simulink model "HVDC_VSC_1CPUcore_dcpl"  (Simulink 8.4)
settings: Solver=ode3  SolverMode=SingleTasking  StartTime=0.0  StopTime=70.0  FixedStep=Ts_Power  RelTol=1e-3  AbsTol=1e-2
PreLoadFcn:
  | Ts_Power=50e-6; Ts_Control=1*Ts_Power; init_cosim_IA; startup_transients_hvdc_vsc;
PostLoadFcn:
  | Ts_Power=50e-6; Ts_Control=1*Ts_Power; init_cosim_IA; startup_transients_hvdc_vsc;
InitFcn:
  | Ts_Power=50e-6; Ts_Control=1*Ts_Power; init_cosim_IA; startup_transients_hvdc_vsc;
values from neighbouring files (symbols this model uses):
  dPref1_2 = 0.125    [startup_transients_hvdc_vsc.m]
  dPref1_2_rlimit = 0.6    [startup_transients_hvdc_vsc.m]
  t_deblock_Pref1 = 0.5    [startup_transients_hvdc_vsc.m]
  t_deblock_Udref2 = 0.3    [startup_transients_hvdc_vsc.m]
  t_dPref1_2 = 25.0    (= 25)    [startup_transients_hvdc_vsc.m]
  t_SwitchITMIdc = 0.2    [startup_transients_hvdc_vsc.m]
  t_SwitchITMVdc = 0.1    [startup_transients_hvdc_vsc.m]
undefined symbols (not defined in the file or in its folder): CLARK, D1, Delta, gcbh, h, intfDelay, level, lib_mesures, magnitude, ResistanceM, rte_drive_private_lib, rte_tsb3level_hiz_rect_cb, sps_rtmsupport, Ts_intf, TSB3_hiZR
libraries: powerlib x183, spsVIMeasurementModel x102, powerlib_extras x71, powerlib_meascontrol x50, rteventslib x26, op_dpl_lib x20, rtlab x12, sps_avr x6, artemis x1
(part 1 of 13)
Description:
  | The 'Model  initialization function' defined in the
  | 
  | Model Properties automatically sets the sample time
  | 
  | Ts to 50e-6 s
settings Model: ARTEMISmethode_block_infos=$$__separator__$$HVDC_VSC_1CPUcore_dcpl/ARTEMIS Guide$$__separator__$$  Creator=Gilbert Sybille, IREQ  LastModifiedBy=marij  CovSFcnEnable=on  ExtModeTrigMode=oneshot  ExtModeArmWhenConnect=off  ExtModeAutoUpdateStatusClock=off  BufferReuse=off
settings DataIOCC: LimitDataPoints=off  SaveFormat=StructureWithTime  SaveOutput=off  DSMLogging=off  SaveTime=off  SignalLoggingName=sigsOut
settings OptimizationCC: BlockReduction=off  BooleanDataType=off  OptimizeBlockIOStorage=off  BufferReuse=off  GlobalBufferReuse=off  ExpressionFolding=off  LocalBlockOutputs=off  InitFltsAndDblsToZero=on
settings DebuggingCC: SaveWithParameterizedLinksMsg=none  CheckExecutionContextPreStartOutputMsg=on  CheckExecutionContextRuntimeOutputMsg=on  SignalResolutionControl=TryResolveAllWithWarning  SolverPrmCheckMsg=none  MultiTaskDSMMsg=warning  MultiTaskCondExecSysMsg=none  FcnCallInpInsideContextMsg=EnableAllAsWarning  UnconnectedInputMsg=none  UnconnectedOutputMsg=none  UnconnectedLineMsg=none  FrameProcessingCompatibilityMsg=error
settings HardwareCC: TargetHWDeviceType=32-bit Generic  ProdEqTarget=off
settings GRTTargetCC: TargetFcnLib=ansi_tfl_tmw.mat

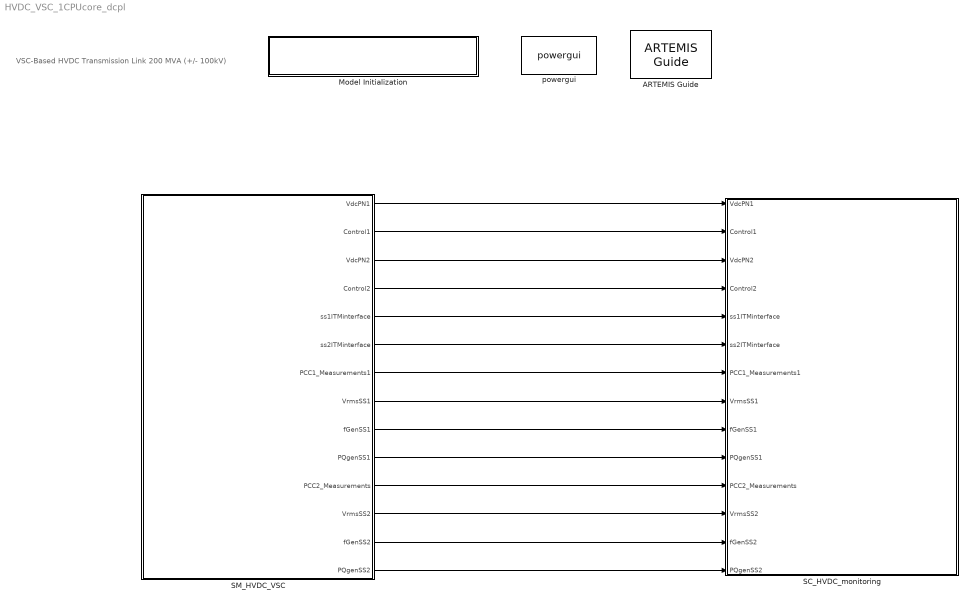
== system HVDC_VSC_1CPUcore_dcpl ==
  note: VSC-Based HVDC Transmission Link
      | 200 MVA  (+/- 100kV)
  ARTEMIS Guide : artemis/ARTEMIS/ARTEMIS Guide  Tag=FTSSmethode_opal_4hx0r99  Description=5.0_z1  lock=on  Ts=Ts_Power  opt=art5  dyna=off  nb_perm=4  RT_fullcomp=off  ssn=off  ssn_itvc=off  ssn_ivic=off  ssn_ext=off  ssn_solver=Trapezoidal  ssn_impulse=off  ssn_quasimpulse=off  ssn_impulse_loop=5  paraExtinctionThy=off  Thy_Impulse=on  dtc=Off  dtc_opt=normal  ao=on  simtype=off  ct_mac=off  lin_mov=off  lsp=[0.001 2]  spike_skip=Disabled  dtc_extra=1  dtc_sws=normal  dtc_pied=0.5  SPSRulesBlock=SPSRules  tre=on  ctmm=off  LF=off  dpl_type=ARTEMiS DPL  rlc_type=off  custom_type=off  para=on  ssn_ImpulseLoopBlockedStateUpdate=5  ssn_mov_iter_number=5  ssn_switch_iter_number=5
  Model Initialization : Subsystem  mask(Model Functions){InitFcnX=Ts_Power=50e-6; Ts_Control=1*Ts_Power; init_cosim_IA; startup_transients_hvdc_vsc;, prel=on, posl=on, inif=on, strf=off}
      mask prompts: InitFcnX "Initialisation"; prel "Preload Function"; posl "PostLoad Function"; inif "InitFcn"; strf "StartFcn"
      mask init:
      | currentBlock = gcb;
      | root = bdroot(currentBlock);
      | 
      | if ~strcmp(get_param(root,'BlockDiagramType'),'library')
      |     if prel==1
      |         set_param(root, 'PreLoadFcn', InitFcnX);
      |     else
      |         set_param(root, 'PreLoadFcn', '');
      |     end
      |     if inif==1
      |         set_param(root, 'InitFcn', InitFcnX);
      |     else
      |         set_param(root, 'InitFcn', '');
      |     end
      |     if strf==1
      |         set_param(root, 'StartFcn', InitFcnX);
      |     else
      |         set_param(root, 'StartFcn', '');
      |     end
      |     if posl==1
      |         set_param(root, 'PostLoadFcn', InitFcnX);
      |     else
      |         set_param(root, 'PostLoadFcn', '');
      |     end
      | end
      | 
      | pos = get_param(currentBlock, 'Position');
      | width = pos(3) - pos(1); height = pos(4) - pos(2);
      | txt = [ upper(root) '\n' '- InitFcn. . . . . '  get_param(root, 'InitFcn') ];
      settings: CopyFcn=set_param(gcb,'LinkStatus','none')
      mask Display: text(5, height*0.5, txt, 'horizontalAlignment', 'left', 'verticalAlignment', 'middle') ;
  SC_HVDC_monitoring : Subsystem
  SM_HVDC_VSC : Subsystem
  powergui : powerlib/powergui  Priority=2  SimulationMode=Discrete  SolverType=Tustin  SampleTime=Ts_Power  frequency=60  SPID=off  DisableSnubberDevices=off  DisableRonSwitches=off  DisableVfSwitches=off  SwTol=0  DisplayEquations=off  Interpol=off  methode=off  Ts=0  frequencyindice=0  Pbase=100e6  ErrMax=1e-4  Iterations=50  UnitsV=kV  UnitsW=MW  FunctionMessages=off  echomessages=on  HookPort=off  EnableUseOfTLC=off  x0status=zero  RestoreLinks=warning  ResistiveCurrentMeasurement=off  Frange=[0:2:500]  Ylog=off  Xlog=on  ShowGrid=off  save=off  variable=ZData  structure=res_fft  ZoomFFT=on  StartTime=1.5  cycles=2  DisplayStyle=1  fundamental=50  FreqAxis=off  MaxFrequency=3000  frequencyindicesteady=1  RmsSteady=1  display=off
  wires:
  SM_HVDC_VSC/1(VdcPN1) -> SC_HVDC_monitoring/1(VdcPN1)
  SM_HVDC_VSC/2(Control1) -> SC_HVDC_monitoring/2(Control1)
  SM_HVDC_VSC/3(VdcPN2) -> SC_HVDC_monitoring/3(VdcPN2)
  SM_HVDC_VSC/4(Control2) -> SC_HVDC_monitoring/4(Control2)
  SM_HVDC_VSC/5(ss1ITMinterface) -> SC_HVDC_monitoring/5(ss1ITMinterface)
  SM_HVDC_VSC/6(ss2ITMinterface) -> SC_HVDC_monitoring/6(ss2ITMinterface)
  SM_HVDC_VSC/11(PCC2_Measurements) -> SC_HVDC_monitoring/11(PCC2_Measurements)
  SM_HVDC_VSC/13(fGenSS2) -> SC_HVDC_monitoring/13(fGenSS2)
  SM_HVDC_VSC/7(PCC1_Measurements1) -> SC_HVDC_monitoring/7(PCC1_Measurements1)
  SM_HVDC_VSC/8(VrmsSS1) -> SC_HVDC_monitoring/8(VrmsSS1)
  SM_HVDC_VSC/14(PQgenSS2) -> SC_HVDC_monitoring/14(PQgenSS2)
  SM_HVDC_VSC/10(PQgenSS1) -> SC_HVDC_monitoring/10(PQgenSS1)
  SM_HVDC_VSC/9(fGenSS1) -> SC_HVDC_monitoring/9(fGenSS1)
  SM_HVDC_VSC/12(VrmsSS2) -> SC_HVDC_monitoring/12(VrmsSS2)

== system HVDC_VSC_1CPUcore_dcpl/Model Initialization ==

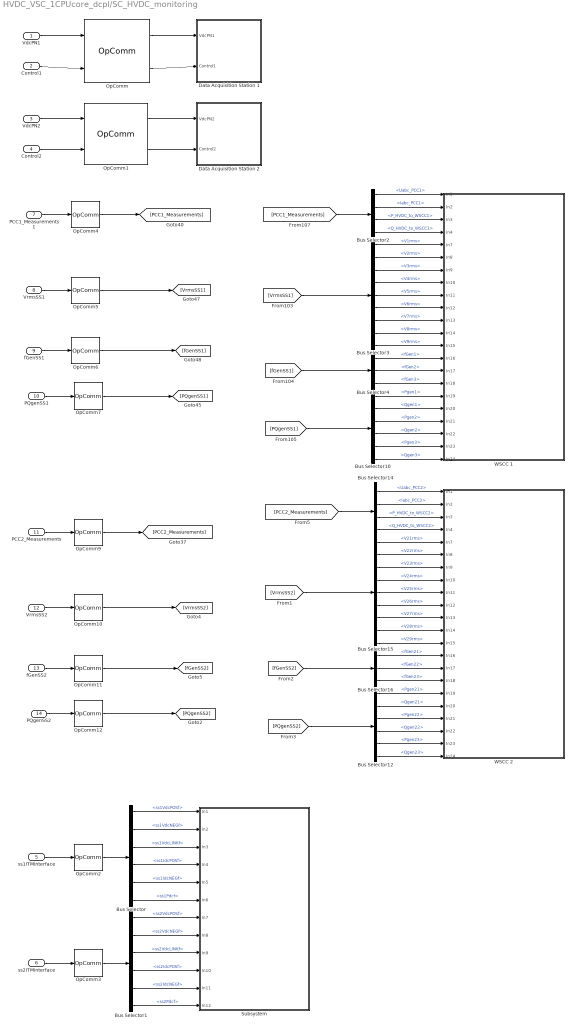
== system HVDC_VSC_1CPUcore_dcpl/SC_HVDC_monitoring ==
  VdcPN1 : Inport
  Control1 : Inport  Port=2
  VdcPN2 : Inport  Port=3
  Control2 : Inport  Port=4
  ss1ITMinterface : Inport  Port=5
  ss2ITMinterface : Inport  Port=6
  PCC1_Measurements1 : Inport  Port=7
  VrmsSS1 : Inport  Port=8
  fGenSS1 : Inport  Port=9
  PQgenSS1 : Inport  Port=10
  PCC2_Measurements : Inport  Port=11
  VrmsSS2 : Inport  Port=12
  fGenSS2 : Inport  Port=13
  PQgenSS2 : Inport  Port=14
  Bus Selector : BusSelector  OutputSignals=ss1VdcPOSf,ss1VdcNEGf,ss1VdcLINKf,ss1IdcPOSf,ss1IdcNEGf,ss1Pdcf
  Bus Selector1 : BusSelector  OutputSignals=ss2VdcPOSf,ss2VdcNEGf,ss2VdcLINKf,ss2IdcPOSf,ss2IdcNEGf,ss2Pdcf
  Bus Selector10 : BusSelector  OutputSignals=Pgen1,Qgen1,Pgen2,Qgen2,Pgen3,Qgen3
  Bus Selector12 : BusSelector  OutputSignals=Pgen21,Qgen21,Pgen22,Qgen22,Pgen23,Qgen23
  Bus Selector14 : BusSelector  OutputSignals=Uabc_PCC2,Iabc_PCC2,P_HVDC_to_WSCC2,Q_HVDC_to_WSCC2
  Bus Selector15 : BusSelector  OutputSignals=V21rms,V22rms,V23rms,V24rms,V25rms,V26rms,V27rms,V28rms,V29rms
  Bus Selector16 : BusSelector  OutputSignals=fGen21,fGen22,fGen23
  Bus Selector2 : BusSelector  OutputSignals=Uabc_PCC1,Iabc_PCC1,P_HVDC_to_WSCC1,Q_HVDC_to_WSCC1
  Bus Selector3 : BusSelector  OutputSignals=V1rms,V2rms,V3rms,V4rms,V5rms,V6rms,V7rms,V8rms,V9rms
  Bus Selector4 : BusSelector  OutputSignals=fGen1,fGen2,fGen3
  Data Acquisition Station 1 : Subsystem
      mask Display: disp('Open this block\nto visualize\nrecorded signals')
  Data Acquisition Station 2 : Subsystem
      mask Display: disp('Open this block\nto visualize\nrecorded signals')
  OpComm : rtlab/OpComm  nbport=2  groupe_acq=1  subsys_rate=Ts_Power  st=0  Synchronization=on  Interpolation=on  Threshold=1.0  Missed_Data=off  Sim_Time=off  Samples=off  dynSigOut=off  from_console=0  warning_done=off  writeOpCommFile=off  Offset=off
  OpComm1 : rtlab/OpComm  nbport=2  groupe_acq=2  subsys_rate=Ts_Power  st=0  Synchronization=on  Interpolation=on  Threshold=1.0  Missed_Data=off  Sim_Time=off  Samples=off  dynSigOut=off  from_console=0  warning_done=off  writeOpCommFile=off  Offset=off
  OpComm10 : rtlab/OpComm  nbport=1  groupe_acq=10  subsys_rate=Ts_Power  st=0  Synchronization=on  Interpolation=on  Threshold=1.0  Missed_Data=off  Sim_Time=off  Samples=off  dynSigOut=off  from_console=0  warning_done=off  writeOpCommFile=off  Offset=off
  OpComm11 : rtlab/OpComm  nbport=1  groupe_acq=11  subsys_rate=Ts_Power  st=0  Synchronization=on  Interpolation=on  Threshold=1.0  Missed_Data=off  Sim_Time=off  Samples=off  dynSigOut=off  from_console=0  warning_done=off  writeOpCommFile=off  Offset=off
  OpComm12 : rtlab/OpComm  nbport=1  groupe_acq=12  subsys_rate=Ts_Power  st=0  Synchronization=on  Interpolation=on  Threshold=1.0  Missed_Data=off  Sim_Time=off  Samples=off  dynSigOut=off  from_console=0  warning_done=off  writeOpCommFile=off  Offset=off
  OpComm2 : rtlab/OpComm  nbport=1  groupe_acq=3  subsys_rate=Ts_Power  st=0  Synchronization=on  Interpolation=on  Threshold=1.0  Missed_Data=off  Sim_Time=off  Samples=off  dynSigOut=off  from_console=0  warning_done=off  writeOpCommFile=off  Offset=off
  OpComm3 : rtlab/OpComm  nbport=1  groupe_acq=4  subsys_rate=Ts_Power  st=0  Synchronization=on  Interpolation=on  Threshold=1.0  Missed_Data=off  Sim_Time=off  Samples=off  dynSigOut=off  from_console=0  warning_done=off  writeOpCommFile=off  Offset=off
  OpComm4 : rtlab/OpComm  nbport=1  groupe_acq=5  subsys_rate=Ts_Power  st=0  Synchronization=on  Interpolation=on  Threshold=1.0  Missed_Data=off  Sim_Time=off  Samples=off  dynSigOut=off  from_console=0  warning_done=off  writeOpCommFile=off  Offset=off
  OpComm5 : rtlab/OpComm  nbport=1  groupe_acq=6  subsys_rate=Ts_Power  st=0  Synchronization=on  Interpolation=on  Threshold=1.0  Missed_Data=off  Sim_Time=off  Samples=off  dynSigOut=off  from_console=0  warning_done=off  writeOpCommFile=off  Offset=off
  OpComm6 : rtlab/OpComm  nbport=1  groupe_acq=7  subsys_rate=Ts_Power  st=0  Synchronization=on  Interpolation=on  Threshold=1.0  Missed_Data=off  Sim_Time=off  Samples=off  dynSigOut=off  from_console=0  warning_done=off  writeOpCommFile=off  Offset=off
  OpComm7 : rtlab/OpComm  nbport=1  groupe_acq=8  subsys_rate=Ts_Power  st=0  Synchronization=on  Interpolation=on  Threshold=1.0  Missed_Data=off  Sim_Time=off  Samples=off  dynSigOut=off  from_console=0  warning_done=off  writeOpCommFile=off  Offset=off
  OpComm9 : rtlab/OpComm  nbport=1  groupe_acq=9  subsys_rate=Ts_Power  st=0  Synchronization=on  Interpolation=on  Threshold=1.0  Missed_Data=off  Sim_Time=off  Samples=off  dynSigOut=off  from_console=0  warning_done=off  writeOpCommFile=off  Offset=off
  Subsystem : Subsystem
  WSCC 1 : Subsystem
  WSCC 2 : Subsystem
  wires:
  VdcPN1/1 -> OpComm/1
  Control1/1 -> OpComm/2
  OpComm/1 -> Data Acquisition Station 1/1(VdcPN1)
  OpComm/2 -> Data Acquisition Station 1/2(Control1)
  VdcPN2/1 -> OpComm1/1
  Control2/1 -> OpComm1/2
  OpComm1/1 -> Data Acquisition Station 2/1(VdcPN2)
  OpComm1/2 -> Data Acquisition Station 2/2(Control2)
  ss1ITMinterface/1 -> OpComm2/1
  OpComm2/1 -> Bus Selector/1
  ss2ITMinterface/1 -> OpComm3/1
  OpComm3/1 -> Bus Selector1/1
  Bus Selector/1 -> Subsystem/1(In1)  "<ss1VdcPOSf>"
  Bus Selector/2 -> Subsystem/2(In2)  "<ss1VdcNEGf>"
  Bus Selector/3 -> Subsystem/3(In3)  "<ss1VdcLINKf>"
  Bus Selector/4 -> Subsystem/4(In4)  "<ss1IdcPOSf>"
  Bus Selector/5 -> Subsystem/5(In5)  "<ss1IdcNEGf>"
  Bus Selector/6 -> Subsystem/6(In6)  "<ss1Pdcf>"
  Bus Selector1/1 -> Subsystem/7(In7)  "<ss2VdcPOSf>"
  Bus Selector1/2 -> Subsystem/8(In8)  "<ss2VdcNEGf>"
  Bus Selector1/3 -> Subsystem/9(In9)  "<ss2VdcLINKf>"
  Bus Selector1/4 -> Subsystem/10(In10)  "<ss2IdcPOSf>"
  Bus Selector1/5 -> Subsystem/11(In11)  "<ss2IdcNEGf>"
  Bus Selector1/6 -> Subsystem/12(In12)  "<ss2Pdcf>"
  [PCC1_Measurements] -> Bus Selector2/1
  [VrmsSS1] -> Bus Selector3/1
  [fGenSS1] -> Bus Selector4/1
  [PQgenSS1] -> Bus Selector10/1
  PCC1_Measurements1/1 -> OpComm4/1
  VrmsSS1/1 -> OpComm5/1
  fGenSS1/1 -> OpComm6/1
  PQgenSS1/1 -> OpComm7/1
  OpComm4/1 -> [PCC1_Measurements]
  OpComm5/1 -> [VrmsSS1]
  OpComm6/1 -> [fGenSS1]
  OpComm7/1 -> [PQgenSS1]
  Bus Selector2/1 -> WSCC 1/1(In1)  "<Uabc_PCC1>"
  Bus Selector2/2 -> WSCC 1/2(In2)  "<Iabc_PCC1>"
  Bus Selector2/3 -> WSCC 1/3(In3)  "<P_HVDC_to_WSCC1>"
  Bus Selector2/4 -> WSCC 1/4(In4)  "<Q_HVDC_to_WSCC1>"
  Bus Selector3/1 -> WSCC 1/5(In7)  "<V1rms>"
  Bus Selector3/2 -> WSCC 1/6(In8)  "<V2rms>"
  Bus Selector3/3 -> WSCC 1/7(In9)  "<V3rms>"
  Bus Selector3/4 -> WSCC 1/8(In10)  "<V4rms>"
  Bus Selector3/5 -> WSCC 1/9(In11)  "<V5rms>"
  Bus Selector3/6 -> WSCC 1/10(In12)  "<V6rms>"
  Bus Selector3/7 -> WSCC 1/11(In13)  "<V7rms>"
  Bus Selector3/8 -> WSCC 1/12(In14)  "<V8rms>"
  Bus Selector3/9 -> WSCC 1/13(In15)  "<V9rms>"
  Bus Selector4/1 -> WSCC 1/14(In16)  "<fGen1>"
  Bus Selector4/2 -> WSCC 1/15(In17)  "<fGen2>"
  Bus Selector4/3 -> WSCC 1/16(In18)  "<fGen3>"
  Bus Selector10/1 -> WSCC 1/17(In19)  "<Pgen1>"
  Bus Selector10/2 -> WSCC 1/18(In20)  "<Qgen1>"
  Bus Selector10/3 -> WSCC 1/19(In21)  "<Pgen2>"
  Bus Selector10/4 -> WSCC 1/20(In22)  "<Qgen2>"
  Bus Selector10/5 -> WSCC 1/21(In23)  "<Pgen3>"
  Bus Selector10/6 -> WSCC 1/22(In24)  "<Qgen3>"
  [PCC2_Measurements] -> Bus Selector14/1
  [VrmsSS2] -> Bus Selector15/1
  [fGenSS2] -> Bus Selector16/1
  [PQgenSS2] -> Bus Selector12/1
  PCC2_Measurements/1 -> OpComm9/1
  VrmsSS2/1 -> OpComm10/1
  fGenSS2/1 -> OpComm11/1
  PQgenSS2/1 -> OpComm12/1
  OpComm9/1 -> [PCC2_Measurements]
  OpComm10/1 -> [VrmsSS2]
  OpComm11/1 -> [fGenSS2]
  OpComm12/1 -> [PQgenSS2]
  Bus Selector14/1 -> WSCC 2/1(In1)  "<Uabc_PCC2>"
  Bus Selector14/2 -> WSCC 2/2(In2)  "<Iabc_PCC2>"
  Bus Selector14/3 -> WSCC 2/3(In3)  "<P_HVDC_to_WSCC2>"
  Bus Selector15/2 -> WSCC 2/6(In8)  "<V22rms>"
  Bus Selector15/3 -> WSCC 2/7(In9)  "<V23rms>"
  Bus Selector15/5 -> WSCC 2/9(In11)  "<V25rms>"
  Bus Selector15/7 -> WSCC 2/11(In13)  "<V27rms>"
  Bus Selector15/8 -> WSCC 2/12(In14)  "<V28rms>"
  Bus Selector15/9 -> WSCC 2/13(In15)  "<V29rms>"
  Bus Selector16/1 -> WSCC 2/14(In16)  "<fGen21>"
  Bus Selector16/2 -> WSCC 2/15(In17)  "<fGen22>"
  Bus Selector16/3 -> WSCC 2/16(In18)  "<fGen23>"
  Bus Selector12/1 -> WSCC 2/17(In19)  "<Pgen21>"
  Bus Selector12/2 -> WSCC 2/18(In20)  "<Qgen21>"
  Bus Selector12/3 -> WSCC 2/19(In21)  "<Pgen22>"
  Bus Selector12/4 -> WSCC 2/20(In22)  "<Qgen22>"
  Bus Selector12/5 -> WSCC 2/21(In23)  "<Pgen23>"
  Bus Selector12/6 -> WSCC 2/22(In24)  "<Qgen23>"
  Bus Selector15/4 -> WSCC 2/8(In10)  "<V24rms>"
  Bus Selector15/6 -> WSCC 2/10(In12)  "<V26rms>"
  Bus Selector14/4 -> WSCC 2/4(In4)  "<Q_HVDC_to_WSCC2>"
  Bus Selector15/1 -> WSCC 2/5(In7)  "<V21rms>"

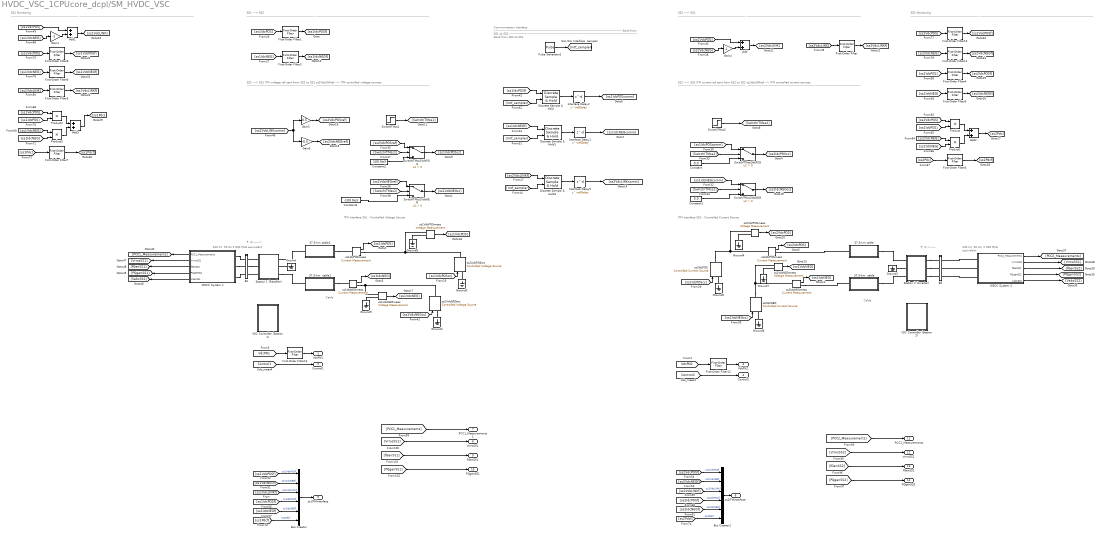
== system HVDC_VSC_1CPUcore_dcpl/SM_HVDC_VSC ==
  note: 230 kV, 50 Hz
      |  2 000 MVA equivalent
  note: P, Q
      | <------
  note: P, Q
      | ------>
  note: Cable
  note: 230 kV, 50 Hz,
      | 2 000 MVA equivalent
  note: Cable
  note: SS2 ---> SS1
      | ITM voltage ref sent from SS2 to SS1
      | ss2VdcLINKref
      | --> ITM controlled voltage sources
      | ------------------------------------------------------------------------------------------------------------------------------------------------------------------------------------
  note: Communication Interface
      |
      | --------------------------------------------------------------------------------------------------------------------------------
      | Send from SS1 to SS2
      |
      | --------------------------------------------------------------------------------------------------------------------------------
      | Send from SS2 to SS1
  note: SS1 ---> SS2
      | ------------------------------------------------------------------------------------------------------------------------------------------------------------------------------------
  note: SS2 ---> SS1
      | ------------------------------------------------------------------------------------------------------------------------------------------------------------------------------------
  note: SS1 ---> SS2
      | ITM current ref sent from SS1 to SS2
      | ss1IdcLINKref
      | --> ITM controlled current sources
      | ------------------------------------------------------------------------------------------------------------------------------------------------------------------------------------
  note: ITM Interface SS1 - Controlled Voltage Source
  note: ITM Interface SS2 - Controlled Current Source
  note: SS1 Monitoring
      | ------------------------------------------------------------------------------------------------------------------------------------------------------------------------------------
  note: SS2 Monitoring
      | ------------------------------------------------------------------------------------------------------------------------------------------------------------------------------------
  37.5-km  cable : Subsystem  mask(Artemis Distributed Parameters Line){SimulationMode=ARTEMIS model, Phases=1, Frequency=60, Resistance=1.3900e-002, Inductance=1.5900e-004, Capacitance=2.3100e-007, Length=37.5, Measurements=None}
      mask prompts: SimulationMode "Simulation Mode"; Phases "Number of phases N"; Frequency "Frequency used for R L C specification (Hz)"; Resistance "Resistance per unit length (Ohms/km)   [N*N matrix] or [R1 R0 R0m]"; Inductance "Inductance per unit length (H/km) [N*N matrix ] or [L1 L0 L0m]"; Capacitance "Capacitance per unit length (F/km) [N*N matrix] or [C1 C0 C0m]"; Length "Line length (km)"
      mask help:
      | Implements a N-phases distributed parameter line model. The R,L, and C line parameters are specified by [NxN] matrices.
      |
      | To model a two-, three-, or a six-phase symetrical line you can either specify complete [NxN] matrices or simply enter sequence parameters vectors: the  positive and zero sequence parameters for a two-phase or  three-phase transposed  line, plus the mutual zero-sequence for a  six-phase transposed  line  (2 coupled 3-phase lines).
      mask init:
      | % Get current block
      | currentBlock = gcb;
      | 
      | % Get electric variables
      | [Zm,R,v,Ti,to,Rt4,h,Zimp,Zmat,Yphase,ResistanceM] = op_distributedparametersline_cb(gcb,'variable_mask_maskinitialization', Phases, Frequency, Resistance, Inductance, Capacitance, Length);
      | 
      | % Set block contents
      | op_distributedparametersline_cb(currentBlock,'maskinitialization');
      mask Help: eval('fts2help(''distributedparametersline'');');
      mask TypeOptions SimulationMode: SimPowerSystems model | ARTEMIS model
      mask TypeOptions Phases: 1 | 2 | 3 | 4 | 5 | 6
      mask TypeOptions Measurements: None
      mask Display:
      | patch([0 0.5 0.7 0],[1 1 0 0],[0.7 0.75 0.9]);
      | patch([1 0.53 0.73 1],[1 1 0 0],[1 0.8 0.7]);
      | plot([0 0 1 1 0],[0 1 1 0 0]);
      | plot([0 0.2 0.2 0.8 0.8 1 0.8 0.8 0.2 0.2 NaN 0 NaN 1],[0.5 0.5 0.625 0.625 0.5 0.5 0.5 0.375 0.375 0.5 NaN 0 NaN 1])
      | disp('DPL')
  37.5-km  cable1 : Subsystem  mask(Artemis Distributed Parameters Line){SimulationMode=ARTEMIS model, Phases=1, Frequency=60, Resistance=1.3900e-002, Inductance=1.5900e-004, Capacitance=2.3100e-007, Length=37.5, Measurements=None}
      mask prompts: SimulationMode "Simulation Mode"; Phases "Number of phases N"; Frequency "Frequency used for R L C specification (Hz)"; Resistance "Resistance per unit length (Ohms/km)   [N*N matrix] or [R1 R0 R0m]"; Inductance "Inductance per unit length (H/km) [N*N matrix ] or [L1 L0 L0m]"; Capacitance "Capacitance per unit length (F/km) [N*N matrix] or [C1 C0 C0m]"; Length "Line length (km)"
      mask help:
      | Implements a N-phases distributed parameter line model. The R,L, and C line parameters are specified by [NxN] matrices.
      |
      | To model a two-, three-, or a six-phase symetrical line you can either specify complete [NxN] matrices or simply enter sequence parameters vectors: the  positive and zero sequence parameters for a two-phase or  three-phase transposed  line, plus the mutual zero-sequence for a  six-phase transposed  line  (2 coupled 3-phase lines).
      mask init: same as HVDC_VSC_1CPUcore_dcpl/SM_HVDC_VSC/37.5-km  cable
      mask Help: eval('fts2help(''distributedparametersline'');');
      mask TypeOptions SimulationMode: SimPowerSystems model | ARTEMIS model
      mask TypeOptions Phases: 1 | 2 | 3 | 4 | 5 | 6
      mask TypeOptions Measurements: None
      mask Display:
      | patch([0 0.5 0.7 0],[1 1 0 0],[0.7 0.75 0.9]);
      | patch([1 0.53 0.73 1],[1 1 0 0],[1 0.8 0.7]);
      | plot([0 0 1 1 0],[0 1 1 0 0]);
      | plot([0 0.2 0.2 0.8 0.8 1 0.8 0.8 0.2 0.2 NaN 0 NaN 1],[0.5 0.5 0.625 0.625 0.5 0.5 0.5 0.375 0.375 0.5 NaN 0 NaN 1])
      | disp('DPL')
  37.5-km cable : Subsystem  mask(Artemis Distributed Parameters Line){SimulationMode=ARTEMIS model, Phases=1, Frequency=60, Resistance=1.3900e-002, Inductance=1.5900e-004, Capacitance=2.3100e-007, Length=37.5, Measurements=None}
      mask prompts: SimulationMode "Simulation Mode"; Phases "Number of phases N"; Frequency "Frequency used for R L C specification (Hz)"; Resistance "Resistance per unit length (Ohms/km)   [N*N matrix] or [R1 R0 R0m]"; Inductance "Inductance per unit length (H/km) [N*N matrix ] or [L1 L0 L0m]"; Capacitance "Capacitance per unit length (F/km) [N*N matrix] or [C1 C0 C0m]"; Length "Line length (km)"
      mask help:
      | Implements a N-phases distributed parameter line model. The R,L, and C line parameters are specified by [NxN] matrices.
      |
      | To model a two-, three-, or a six-phase symetrical line you can either specify complete [NxN] matrices or simply enter sequence parameters vectors: the  positive and zero sequence parameters for a two-phase or  three-phase transposed  line, plus the mutual zero-sequence for a  six-phase transposed  line  (2 coupled 3-phase lines).
      mask init: same as HVDC_VSC_1CPUcore_dcpl/SM_HVDC_VSC/37.5-km  cable
      mask Help: eval('fts2help(''distributedparametersline'');');
      mask TypeOptions SimulationMode: SimPowerSystems model | ARTEMIS model
      mask TypeOptions Phases: 1 | 2 | 3 | 4 | 5 | 6
      mask TypeOptions Measurements: None
      mask Display:
      | patch([0 0.5 0.7 0],[1 1 0 0],[0.7 0.75 0.9]);
      | patch([1 0.53 0.73 1],[1 1 0 0],[1 0.8 0.7]);
      | plot([0 0 1 1 0],[0 1 1 0 0]);
      | plot([0 0.2 0.2 0.8 0.8 1 0.8 0.8 0.2 0.2 NaN 0 NaN 1],[0.5 0.5 0.625 0.625 0.5 0.5 0.5 0.375 0.375 0.5 NaN 0 NaN 1])
      | disp('DPL')
  37.5-km cable1 : Subsystem  mask(Artemis Distributed Parameters Line){SimulationMode=ARTEMIS model, Phases=1, Frequency=60, Resistance=1.3900e-002, Inductance=1.5900e-004, Capacitance=2.3100e-007, Length=37.5, Measurements=None}
      mask prompts: SimulationMode "Simulation Mode"; Phases "Number of phases N"; Frequency "Frequency used for R L C specification (Hz)"; Resistance "Resistance per unit length (Ohms/km)   [N*N matrix] or [R1 R0 R0m]"; Inductance "Inductance per unit length (H/km) [N*N matrix ] or [L1 L0 L0m]"; Capacitance "Capacitance per unit length (F/km) [N*N matrix] or [C1 C0 C0m]"; Length "Line length (km)"
      mask help:
      | Implements a N-phases distributed parameter line model. The R,L, and C line parameters are specified by [NxN] matrices.
      |
      | To model a two-, three-, or a six-phase symetrical line you can either specify complete [NxN] matrices or simply enter sequence parameters vectors: the  positive and zero sequence parameters for a two-phase or  three-phase transposed  line, plus the mutual zero-sequence for a  six-phase transposed  line  (2 coupled 3-phase lines).
      mask init: same as HVDC_VSC_1CPUcore_dcpl/SM_HVDC_VSC/37.5-km  cable
      mask Help: eval('fts2help(''distributedparametersline'');');
      mask TypeOptions SimulationMode: SimPowerSystems model | ARTEMIS model
      mask TypeOptions Phases: 1 | 2 | 3 | 4 | 5 | 6
      mask TypeOptions Measurements: None
      mask Display:
      | patch([0 0.5 0.7 0],[1 1 0 0],[0.7 0.75 0.9]);
      | patch([1 0.53 0.73 1],[1 1 0 0],[1 0.8 0.7]);
      | plot([0 0 1 1 0],[0 1 1 0 0]);
      | plot([0 0.2 0.2 0.8 0.8 1 0.8 0.8 0.2 0.2 NaN 0 NaN 1],[0.5 0.5 0.625 0.625 0.5 0.5 0.5 0.375 0.375 0.5 NaN 0 NaN 1])
      | disp('DPL')
  Add{,1..3} (4 alike) : Sum
  B1 : Subsystem  DialogController=POWERSYS.PowerSysDialog  LoadFcn=sps_rtmsupport('LoadFcn',gcbh);  StartFcn=sps_rtmsupport('StartFcn',gcbh);  StopFcn=sps_rtmsupport('StopFcn',gcbh);  mask(Three-Phase VI Measurement){VoltageMeasurement=phase-to-ground, SetLabelV=on, LabelV=Uabc_B1, Vpu=on, VpuLL=off, CurrentMeasurement=yes, SetLabelI=on, LabelI=Iabc_B1, Ipu=on, Pbase=200e6, Vbase=230e3, OutputType=Magnitude, PhasorSimulation=off, PSBequivalent=0}
      mask prompts: VoltageMeasurement "Voltage measurement"; SetLabelV "Use a label"; LabelV "Signal label  (use a From block to collect this signal)"; Vpu "Voltages in pu,  based on peak value of nominal phase-to-ground voltage"; VpuLL "Voltages in pu,  based on peak value of nominal phase-to-phase  voltage"; CurrentMeasurement "Current measurement"; SetLabelI "Use a label"; LabelI "Signal label  (use a From block to collect this signal)"; Ipu "Currents in pu"; Pbase "Base power ( VA 3 phase)"; Vbase "Nominal voltage used for pu measurement (Vrms phase-phase) :"; OutputType "Output signals in:"; PhasorSimulation "Phasor simulation (internal use)"; PSBequivalent "Equivalent circuit (internal use)"
      mask help:
      | Ideal three-phase voltage and current measurements.
      |
      | The block can output the voltages and currents in per unit values or in volts and amperes.
      mask init:
      | block = gcb;
      | Kv=1;
      | Ki=1;
      | [Kv,Ki] = powericon('ThreePhaseVIMeasurementParam',block,Vpu,VpuLL,Ipu,Vbase,Pbase,PhasorSimulation,OutputType);
      | powericon('ThreePhaseVIMeasurementCback',block);
      | power_initmask();
      settings: CopyFcn=sps_rtmsupport('CopyFcn',gcbh); powericon('ThreePhaseVIMeasurementCopy',gcb)  DeleteFcn=sps_rtmsupport('DeleteFcn',gcbh);  UndoDeleteFcn=sps_rtmsupport('UndoDeleteFcn',gcbh);  ModelCloseFcn=sps_rtmsupport('ModelCloseFcn',gcbh);  PreSaveFcn="sps_rtmsupport('PreSaveFcn',gcbh);  set_param(gcb,'LinkStatus','restore')"  PostSaveFcn=sps_rtmsupport('PostSaveFcn',gcbh);  NameChangeFcn=sps_rtmsupport('NameChangeFcn',gcbh);  PreCopyFcn=sps_rtmsupport('PreCopyFcn',gcbh);  OpenFcn=sps_rtmsupport('OpenFcn',gcbh, [1 2 4 5 6 7 9 -12 13]);  CloseFcn=sps_rtmsupport('CloseFcn',gcbh);  PreDeleteFcn=sps_rtmsupport('PreDeleteFcn',gcbh);
      mask Help: helpview(psbhelp)
      mask TypeOptions VoltageMeasurement: no | phase-to-ground | phase-to-phase
      mask Callback VoltageMeasurement: powericon('ThreePhaseVIMeasurementCback',gcb,'Vselector');
      mask Callback SetLabelV: powericon('ThreePhaseVIMeasurementCback',gcb,'');
      mask Callback Vpu: powericon('ThreePhaseVIMeasurementCback',gcb,'Vpu');
      mask Callback VpuLL: powericon('ThreePhaseVIMeasurementCback',gcb,'VpuLL');
      mask TypeOptions CurrentMeasurement: no | yes
      mask Callback CurrentMeasurement: powericon('ThreePhaseVIMeasurementCback',gcb,'');
      mask Callback SetLabelI: powericon('ThreePhaseVIMeasurementCback',gcb,'');
      mask Callback LabelI: powericon('ThreePhaseVIMeasurementCback',gcb,'');
      mask Callback Ipu: powericon('ThreePhaseVIMeasurementCback',gcb,'');
      mask TypeOptions OutputType: Complex | Real-Imag | Magnitude-Angle | Magnitude
  B2 : Subsystem  DialogController=POWERSYS.PowerSysDialog  LoadFcn=sps_rtmsupport('LoadFcn',gcbh);  StartFcn=sps_rtmsupport('StartFcn',gcbh);  StopFcn=sps_rtmsupport('StopFcn',gcbh);  mask(Three-Phase VI Measurement){VoltageMeasurement=phase-to-ground, SetLabelV=on, LabelV=Uabc_B2, Vpu=on, VpuLL=off, CurrentMeasurement=yes, SetLabelI=on, LabelI=Iabc_B2, Ipu=on, Pbase=200e6, Vbase=230e3, OutputType=Magnitude, PhasorSimulation=off, PSBequivalent=0}
      mask prompts: VoltageMeasurement "Voltage measurement"; SetLabelV "Use a label"; LabelV "Signal label  (use a From block to collect this signal)"; Vpu "Voltages in pu,  based on peak value of nominal phase-to-ground voltage"; VpuLL "Voltages in pu,  based on peak value of nominal phase-to-phase  voltage"; CurrentMeasurement "Current measurement"; SetLabelI "Use a label"; LabelI "Signal label  (use a From block to collect this signal)"; Ipu "Currents in pu"; Pbase "Base power ( VA 3 phase)"; Vbase "Nominal voltage used for pu measurement (Vrms phase-phase) :"; OutputType "Output signals in:"; PhasorSimulation "Phasor simulation (internal use)"; PSBequivalent "Equivalent circuit (internal use)"
      mask help:
      | Ideal three-phase voltage and current measurements.
      |
      | The block can output the voltages and currents in per unit values or in volts and amperes.
      mask init: same as HVDC_VSC_1CPUcore_dcpl/SM_HVDC_VSC/B1
      settings: CopyFcn=sps_rtmsupport('CopyFcn',gcbh); powericon('ThreePhaseVIMeasurementCopy',gcb)  DeleteFcn=sps_rtmsupport('DeleteFcn',gcbh);  UndoDeleteFcn=sps_rtmsupport('UndoDeleteFcn',gcbh);  ModelCloseFcn=sps_rtmsupport('ModelCloseFcn',gcbh);  PreSaveFcn="sps_rtmsupport('PreSaveFcn',gcbh);  set_param(gcb,'LinkStatus','restore')"  PostSaveFcn=sps_rtmsupport('PostSaveFcn',gcbh);  NameChangeFcn=sps_rtmsupport('NameChangeFcn',gcbh);  PreCopyFcn=sps_rtmsupport('PreCopyFcn',gcbh);  OpenFcn=sps_rtmsupport('OpenFcn',gcbh, [1 2 4 5 6 7 9 -12 13]);  CloseFcn=sps_rtmsupport('CloseFcn',gcbh);  PreDeleteFcn=sps_rtmsupport('PreDeleteFcn',gcbh);
      mask Help: helpview(psbhelp)
      mask TypeOptions VoltageMeasurement: no | phase-to-ground | phase-to-phase
      mask Callback VoltageMeasurement: powericon('ThreePhaseVIMeasurementCback',gcb,'Vselector');
      mask Callback SetLabelV: powericon('ThreePhaseVIMeasurementCback',gcb,'');
      mask Callback Vpu: powericon('ThreePhaseVIMeasurementCback',gcb,'Vpu');
      mask Callback VpuLL: powericon('ThreePhaseVIMeasurementCback',gcb,'VpuLL');
      mask TypeOptions CurrentMeasurement: no | yes
      mask Callback CurrentMeasurement: powericon('ThreePhaseVIMeasurementCback',gcb,'');
      mask Callback SetLabelI: powericon('ThreePhaseVIMeasurementCback',gcb,'');
      mask Callback LabelI: powericon('ThreePhaseVIMeasurementCback',gcb,'');
      mask Callback Ipu: powericon('ThreePhaseVIMeasurementCback',gcb,'');
      mask TypeOptions OutputType: Complex | Real-Imag | Magnitude-Angle | Magnitude
  Bus Creator : BusCreator  Inputs=6
  Bus Creator1 : BusCreator  Inputs=6
  Constant : Constant  Value=0.0
  Constant1 : Constant  Value=0.0
  Constant2 : Constant  Value=100.0e3
  Constant3 : Constant  Value=-100.0e3
  Discrete Sample & Hold : powerlib_extras/Discrete  Control Blocks/Discrete Sample & Hold  ic=0  Ts=Ts_intf
  Discrete Sample & Hold1 : powerlib_extras/Discrete  Control Blocks/Discrete Sample & Hold  ic=0  Ts=Ts_intf
  Discrete Sample & Hold4 : powerlib_extras/Discrete  Control Blocks/Discrete Sample & Hold  ic=0  Ts=Ts_intf
  First-Order Filter{,1..13} (14 alike) : powerlib_meascontrol/Filters/First-Order Filter  FilterType=Lowpass  Tc=0.05  Ts=Ts_Power  Initialize=on  Vac_Init=[0, 0, 0]  Vdc_Init=0  PlotResponse=off  FreqRange="[0,  200,  1]"
  Gain1 : Gain  Gain=-1
  Gain4 : Gain  Gain=-1
  Gain5 : Gain  Gain=0.5
  Gain6 : Gain  Gain=-0.5
  Ground{,1..9} (10 alike) : powerlib/Elements/Ground  LConnTagsString=a
  Interface Delay1 : Delay  DelayLength=intfDelay  InputProcessing=Inherited
  Interface Delay2 : Delay  DelayLength=intfDelay  InputProcessing=Inherited
  Interface Delay5 : Delay  DelayLength=intfDelay  InputProcessing=Inherited
  Product{,1..3} (4 alike) : Product
  Pulse Generator2 : DiscretePulseGenerator  Period=h  SampleTime=Ts_intf
  Station 1 (Rectifier) : Subsystem
  Station 2 (Inverter) : Subsystem
  SwitchITMss1 : Step  Time=t_SwitchITMVdc  SampleTime=Ts_Control
  SwitchITMss1VdcNEG : Switch  Criteria=u2 > Threshold
  SwitchITMss1VdcPOS : Switch  Criteria=u2 > Threshold
  SwitchITMss2 : Step  Time=t_SwitchITMIdc  SampleTime=Ts_Control
  SwitchITMss2IdcNEG : Switch  Criteria=u2 > Threshold
  SwitchITMss2IdcPOS : Switch  Criteria=u2 > Threshold
  VSC Controller (Station 1) : Subsystem
  VSC Controller (Station 2) : Subsystem
  WSCC System 1 : Subsystem
  WSCC System 2 : Subsystem
  ss1IdcNEGmeas : powerlib/Measurements/Current Measurement  PhasorSimulation=off  OutputType=Complex  PSBequivalent=0
  ss1IdcPOSmeas : powerlib/Measurements/Current Measurement  PhasorSimulation=off  OutputType=Complex  PSBequivalent=0
  ss1VdcNEGmeas : powerlib/Measurements/Voltage Measurement  PhasorSimulation=off  OutputType=Complex  PSBequivalent=0
  ss1VdcPOSmeas : powerlib/Measurements/Voltage Measurement  PhasorSimulation=off  OutputType=Complex  PSBequivalent=0
  ss2IdcNEG : powerlib/Electrical Sources/Controlled Current Source  Initialize=on  Source_Type=DC  Amplitude=0.0  Phase=0  Frequency=0  Measurements=None
  ss2IdcNEGmeas : powerlib/Measurements/Current Measurement  PhasorSimulation=off  OutputType=Complex  PSBequivalent=0
  ss2IdcPOS : powerlib/Electrical Sources/Controlled Current Source  Initialize=on  Source_Type=DC  Amplitude=0.0  Phase=0  Frequency=0  Measurements=None
  ss2IdcPOSmeas : powerlib/Measurements/Current Measurement  PhasorSimulation=off  OutputType=Complex  PSBequivalent=0
  ss2UdcNEGsrc : powerlib/Electrical Sources/Controlled Voltage Source  Initialize=on  Source_Type=DC  Amplitude=-100.0e3  Phase=0  Frequency=0  Measurements=None
  ss2UdcPOSsrc : powerlib/Electrical Sources/Controlled Voltage Source  Initialize=on  Source_Type=DC  Amplitude=100.0e3  Phase=0  Frequency=0  Measurements=None
  ss2VdcNEGmeas : powerlib/Measurements/Voltage Measurement  PhasorSimulation=off  OutputType=Complex  PSBequivalent=0
  ss2VdcPOSmeas : powerlib/Measurements/Voltage Measurement  PhasorSimulation=off  OutputType=Complex  PSBequivalent=0
  VdcPN1 : Outport
  Control1 : Outport  Port=2
  VdcPN2 : Outport  Port=3
  Control2 : Outport  Port=4
  ss1ITMinterface : Outport  Port=5
  ss2ITMinterface : Outport  Port=6
  PCC1_Measurements1 : Outport  Port=7
  VrmsSS1 : Outport  Port=8
  fGenSS1 : Outport  Port=9
  PQgenSS1 : Outport  Port=10
  PCC2_Measurements : Outport  Port=11
  VrmsSS2 : Outport  Port=12
  fGenSS2 : Outport  Port=13
  PQgenSS2 : Outport  Port=14
  wires:
  [VdcPN1] -> First-Order Filter13/1
  [Control2] -> Control2/1
  [VdcPN2] -> First-Order Filter12/1
  [Control1] -> Control1/1
  ss2VdcNEGmeas/1 -> [ss2VdcNEG]
  ss2VdcPOSmeas/1 -> [ss2VdcPOS]
  ss1IdcPOSmeas/1 -> [ss1IdcPOS]
  ss1IdcNEGmeas/1 -> [ss1IdcNEG]
  [ss2IdcNEGcc] -> ss2IdcNEG/1
  [ss2IdcPOScc] -> ss2IdcPOS/1
  Discrete Sample & Hold/1 -> Interface Delay2/1
  Interface Delay2/1 -> [ss1IdcPOScomm]
  Pulse Generator2/1 -> [Intf_sampler]
  Interface Delay1/1 -> [ss1IdcNEGcomm]
  [Intf_sampler] -> Discrete Sample & Hold1/2
  Discrete Sample & Hold1/1 -> Interface Delay1/1
  SwitchITMss2IdcPOS/1 -> [ss2IdcPOScc]
  Constant/1 -> SwitchITMss2IdcPOS/3
  [SwitchITMss2] -> SwitchITMss2IdcPOS/2
  Constant1/1 -> SwitchITMss2IdcNEG/3
  [SwitchITMss2] -> SwitchITMss2IdcNEG/2
  Constant3/1 -> SwitchITMss1VdcNEG/3
  [ss2VdcNEGref] -> SwitchITMss1VdcNEG/1
  Constant2/1 -> SwitchITMss1VdcPOS/3
  [ss2VdcPOSref] -> SwitchITMss1VdcPOS/1
  SwitchITMss1VdcPOS/1 -> [ss1VdcPOScc]
  [SwitchITMss1] -> SwitchITMss1VdcPOS/2
  [SwitchITMss1] -> SwitchITMss1VdcNEG/2
  [ss1VdcPOScc] -> ss2UdcPOSsrc/1
  [ss1VdcNEGcc] -> ss2UdcNEGsrc/1
  SwitchITMss1/1 -> [SwitchITMss1]
  SwitchITMss2/1 -> [SwitchITMss2]
  ss2IdcPOSmeas/1 -> [ss2IdcPOS]
  ss1VdcPOSmeas/1 -> [ss1VdcPOS]
  ss1VdcNEGmeas/1 -> [ss1VdcNEG]
  Discrete Sample & Hold4/1 -> Interface Delay5/1
  Interface Delay5/1 -> [ss2VdcLINKcomm]
  [ss2VdcNEG] -> Gain4/1
  [ss2VdcPOS] -> Add/1
  Gain4/1 -> Add/2
  [ss2VdcLINKcomm] -> Gain5/1, Gain6/1
  Gain6/1 -> [ss2VdcNEGref]
  Gain5/1 -> [ss2VdcPOSref]
  [ss1IdcPOScomm] -> SwitchITMss2IdcPOS/1
  [ss1IdcNEGcomm] -> SwitchITMss2IdcNEG/1
  ss2IdcNEGmeas/1 -> [ss2IdcNEG]
  [ss1IdcPOS] -> First-Order Filter1/1
  [ss1IdcNEG] -> First-Order Filter2/1
  SwitchITMss2IdcNEG/1 -> [ss2IdcNEGcc]
  SwitchITMss1VdcNEG/1 -> [ss1VdcNEGcc]
  First-Order Filter1/1 -> [ss1IdcPOSf]
  First-Order Filter2/1 -> [ss1IdcNEGf]
  [ss1IdcNEGf] -> Discrete Sample & Hold1/1
  [Intf_sampler] -> Discrete Sample & Hold/2
  [ss1IdcPOSf] -> Discrete Sample & Hold/1
  Add/1 -> [ss2VdcLINK]
  [ss2VdcLINK] -> First-Order Filter/1
  First-Order Filter/1 -> [ss2VdcLINKf]
  [ss2VdcLINKf] -> Discrete Sample & Hold4/1
  [Intf_sampler] -> Discrete Sample & Hold4/2
  [ss1VdcNEG] -> Gain1/1
  [ss1VdcPOS] -> Add1/1
  Gain1/1 -> Add1/2
  Add1/1 -> [ss1VdcLINK]
  [ss1VdcLINK] -> First-Order Filter3/1
  First-Order Filter3/1 -> [ss1VdcLINKf]
  [ss2IdcPOS] -> First-Order Filter4/1
  [ss2IdcNEG] -> First-Order Filter5/1
  First-Order Filter4/1 -> [ss2IdcPOSf]
  First-Order Filter5/1 -> [ss2IdcNEGf]
  [ss2VdcPOS] -> Product/1
  [ss2IdcPOS] -> Product/2
  [ss2VdcNEG] -> Product1/1
  [ss2IdcNEG] -> Product1/2
  Product/1 -> Add2/1
  Product1/1 -> Add2/2
  Add2/1 -> [ss2Pdc]
  [ss2Pdc] -> First-Order Filter6/1
  First-Order Filter6/1 -> [ss2Pdcf]
  [ss1VdcPOS] -> Product2/1
  [ss1IdcPOS] -> Product2/2
  [ss1VdcNEG] -> Product3/1
  [ss1IdcNEG] -> Product3/2
  Product2/1 -> Add3/1
  Product3/1 -> Add3/2
  Add3/1 -> [ss1Pdc]
  [ss1Pdc] -> First-Order Filter7/1
  First-Order Filter7/1 -> [ss1Pdcf]
  [ss1VdcLINKf] -> Bus Creator/3  "ss1VdcLINKf"
  [ss1IdcPOSf] -> Bus Creator/4  "ss1IdcPOSf"
  [ss1IdcNEGf] -> Bus Creator/5  "ss1IdcNEGf"
  [ss1VdcPOSf] -> Bus Creator/1  "ss1VdcPOSf"
  [ss1VdcNEGf] -> Bus Creator/2  "ss1VdcNEGf"
  [ss1Pdcf] -> Bus Creator/6  "ss1Pdcf"
  Bus Creator/1 -> ss1ITMinterface/1
  [ss2VdcLINKf] -> Bus Creator1/3  "ss2VdcLINKf"
  [ss2IdcPOSf] -> Bus Creator1/4  "ss2IdcPOSf"
  [ss2IdcNEGf] -> Bus Creator1/5  "ss2IdcNEGf"
  [ss2VdcPOSf] -> Bus Creator1/1  "ss2VdcPOSf"
  [ss2VdcNEGf] -> Bus Creator1/2  "ss2VdcNEGf"
  [ss2Pdcf] -> Bus Creator1/6  "ss2Pdcf"
  Bus Creator1/1 -> ss2ITMinterface/1
  [ss1VdcPOS] -> First-Order Filter8/1
  First-Order Filter8/1 -> [ss1VdcPOSf]
  [ss1VdcNEG] -> First-Order Filter9/1
  First-Order Filter9/1 -> [ss1VdcNEGf]
  [ss2VdcPOS] -> First-Order Filter10/1
  [ss2VdcNEG] -> First-Order Filter11/1
  First-Order Filter10/1 -> [ss2VdcPOSf]
  First-Order Filter11/1 -> [ss2VdcNEGf]
  WSCC System 2/1(PCC2_Measurements) -> [PCC2_Measurements]
  WSCC System 2/2(VrmsSS2) -> [VrmsSS2]
  WSCC System 2/3(fGenSS2) -> [fGenSS2]
  WSCC System 2/4(PQgenSS2) -> [PQgenSS2]
  WSCC System 2/5(VabcSS2) -> [VabcSS2]
  WSCC System 1/1(PCC1_Measurements) -> [PCC1_Measurements]
  WSCC System 1/2(VrmsSS1) -> [VrmsSS1]
  WSCC System 1/3(fGenSS1) -> [fGenSS1]
  WSCC System 1/4(PQgenSS1) -> [PQgenSS1]
  WSCC System 1/5(VabcSS1) -> [VabcSS1]
  [VrmsSS1] -> VrmsSS1/1
  [PQgenSS1] -> PQgenSS1/1
  [fGenSS1] -> fGenSS1/1
  [PCC1_Measurements] -> PCC1_Measurements1/1
  [PCC2_Measurements] -> PCC2_Measurements/1
  [VrmsSS2] -> VrmsSS2/1
  [fGenSS2] -> fGenSS2/1
  [PQgenSS2] -> PQgenSS2/1
  First-Order Filter12/1 -> VdcPN2/1
  First-Order Filter13/1 -> VdcPN1/1
  connections:
  WSCC System 2/LConn1 -- B2/LConn1
  WSCC System 2/LConn2 -- B2/LConn2
  WSCC System 2/LConn3 -- B2/LConn3
  Station 1 (Rectifier)/LConn1 -- B1/RConn1
  B1/RConn2 -- Station 1 (Rectifier)/LConn2
  Station 1 (Rectifier)/LConn3 -- B1/RConn3
  Station 2 (Inverter)/LConn1 -- B2/RConn1
  Station 2 (Inverter)/LConn2 -- B2/RConn2
  Station 2 (Inverter)/LConn3 -- B2/RConn3
  Ground/LConn1 -- Station 1 (Rectifier)/RConn2
  Ground1/LConn1 -- Station 2 (Inverter)/RConn2
  Ground2/LConn1 -- ss2UdcNEGsrc/LConn1
  ss1IdcPOSmeas/RConn1 -- ss1VdcPOSmeas/LConn1 -- ss2UdcPOSsrc/RConn1
  Ground3/LConn1 -- ss2UdcPOSsrc/LConn1
  ss1IdcNEGmeas/RConn1 -- ss1VdcNEGmeas/LConn1 -- ss2UdcNEGsrc/RConn1
  Ground4/LConn1 -- ss2VdcPOSmeas/LConn2
  Ground5/LConn1 -- ss2IdcPOS/LConn1
  Ground6/LConn1 -- ss2IdcNEG/LConn1
  ss2VdcNEGmeas/LConn2 -- Ground7/LConn1
  ss2IdcNEG/RConn1 -- ss2VdcNEGmeas/LConn1 -- ss2IdcNEGmeas/LConn1
  ss2IdcPOS/RConn1 -- ss2IdcPOSmeas/LConn1 -- ss2VdcPOSmeas/LConn1
  37.5-km cable/RConn1 -- Station 2 (Inverter)/RConn1
  37.5-km  cable/RConn1 -- Station 2 (Inverter)/RConn3
  Station 1 (Rectifier)/RConn1 -- 37.5-km cable1/LConn1
  Station 1 (Rectifier)/RConn3 -- 37.5-km  cable1/LConn1
  ss1VdcPOSmeas/LConn2 -- Ground8/LConn1
  ss1VdcNEGmeas/LConn2 -- Ground9/LConn1
  37.5-km cable1/RConn1 -- ss1IdcPOSmeas/LConn1
  37.5-km  cable1/RConn1 -- ss1IdcNEGmeas/LConn1
  ss2IdcNEGmeas/RConn1 -- 37.5-km  cable/LConn1
  ss2IdcPOSmeas/RConn1 -- 37.5-km cable/LConn1
  WSCC System 1/LConn3 -- B1/LConn3
  WSCC System 1/LConn1 -- B1/LConn1
  WSCC System 1/LConn2 -- B1/LConn2

== system HVDC_VSC_1CPUcore_dcpl/SC_HVDC_monitoring/Data Acquisition Station 1 ==
  VdcPN1 : Inport
  Control1 : Inport  Port=2
  BUS B1 STATION_1 : Scope
      settings: TimeRange=5  YMin=0.2  YMax=1.2  SaveName=res_2a  Decimation=10  SampleTime=Ts_Control
  Bus Selector : BusSelector  OutputSignals=Pdc_meas (pu)
  Bus Selector4 : BusSelector  OutputSignals=P_meas (pu),Pref_ramped (pu)
  DC_SIDE STATION_1 : Scope  NumInputPorts=2
      settings: TimeRange=5  YMin=-150000~0.99  YMax=150000~1  SaveName=ScopeData2  Decimation=10  SampleTime=Ts_Control
  Mux1 : Mux  Inputs=2
  Pdc_meas [p.u] 1 p.u. = 200MW : Display
  pu-->V : Gain  Gain=100e3/sqrt(3)*sqrt(2)
  wires:
  [VdcPN1] -> pu-->V/1  "Vdc PN (pu AC)"
  Bus Selector/1 -> Pdc_meas [p.u] 1 p.u. = 200MW/1, DC_SIDE STATION_1/2  "<Pdc_meas (pu)>"
  [Control1] -> Bus Selector/1
  Bus Selector4/1 -> Mux1/1  "<P_meas (pu)>"
  Bus Selector4/2 -> Mux1/2  "<Pref_ramped (pu)>"
  Mux1/1 -> BUS B1 STATION_1/1  "P_meas  Pref (pu)"
  pu-->V/1 -> DC_SIDE STATION_1/1  "Vdc PN (V)"
  [Control1] -> Bus Selector4/1
  Control1/1 -> [Control1]
  VdcPN1/1 -> [VdcPN1]

== system HVDC_VSC_1CPUcore_dcpl/SC_HVDC_monitoring/Data Acquisition Station 2 ==
  VdcPN2 : Inport
  Control2 : Inport  Port=2
  Bus Selector : BusSelector  OutputSignals=Pdc_meas (pu)
  DC_SIDE STATION_2 : Scope  NumInputPorts=2
      settings: TimeRange=8  YMin=-148523~-0.14852  YMax=148523~1.33672  SaveName=ScopeData2  Decimation=10  SampleTime=Ts_Control
  Pdc_meas [p.u] 1 p.u. = 200MW : Display
  pu-->V : Gain  Gain=100e3/sqrt(3)*sqrt(2)
  wires:
  pu-->V/1 -> DC_SIDE STATION_2/1  "Vdc PN (V)"
  [Control2] -> Bus Selector/1
  Bus Selector/1 -> Pdc_meas [p.u] 1 p.u. = 200MW/1, DC_SIDE STATION_2/2  "<Pdc_meas (pu)>"
  [VdcPN2] -> pu-->V/1  "Vdc PN (pu AC)"
  Control2/1 -> [Control2]
  VdcPN2/1 -> [VdcPN2]

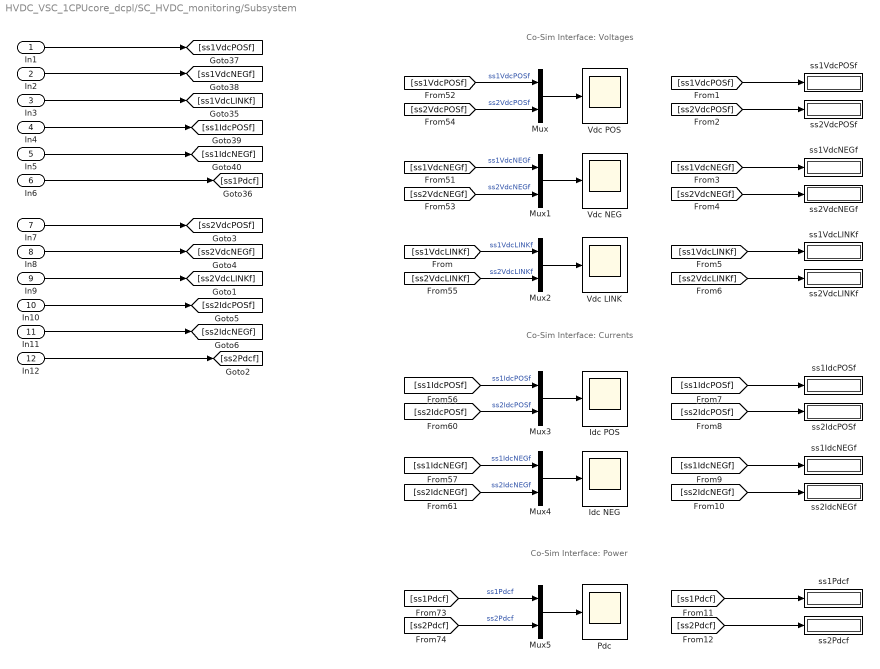
== system HVDC_VSC_1CPUcore_dcpl/SC_HVDC_monitoring/Subsystem ==
  note: Co-Sim Interface: Voltages
  note: Co-Sim Interface: Currents
  note: Co-Sim Interface: Power
  In1 : Inport
  In2 : Inport  Port=2
  In3 : Inport  Port=3
  In4 : Inport  Port=4
  In5 : Inport  Port=5
  In6 : Inport  Port=6
  In7 : Inport  Port=7
  In8 : Inport  Port=8
  In9 : Inport  Port=9
  In10 : Inport  Port=10
  In11 : Inport  Port=11
  In12 : Inport  Port=12
  Idc NEG : Scope
      settings: ShowLegends=on  YMin=-100  YMax=600  SaveName=ScopeData6  Decimation=10  ScrollMode=on
  Idc POS : Scope
      settings: ShowLegends=on  YMin=-600  YMax=100  SaveName=ScopeData5  Decimation=10  ScrollMode=on
  Mux{,1..5} (6 alike) : Mux  Inputs=2
  Pdc : Scope
      settings: ShowLegends=on  YMin=-7e+07  YMax=2e+07  SaveName=ScopeData7  Decimation=10  ScrollMode=on
  Vdc LINK : Scope
      settings: ShowLegends=on  YMin=0  YMax=250000  SaveName=ScopeData3  Decimation=10  ScrollMode=on
  Vdc NEG : Scope
      settings: ShowLegends=on  YMin=-120000  YMax=0  Decimation=10  ScrollMode=on
  Vdc POS : Scope
      settings: ShowLegends=on  YMin=0  YMax=120000  Decimation=10  ScrollMode=on
  ss1IdcNEGf : Display
  ss1IdcPOSf : Display
  ss1Pdcf : Display
  ss1VdcLINKf : Display
  ss1VdcNEGf : Display
  ss1VdcPOSf : Display
  ss2IdcNEGf : Display
  ss2IdcPOSf : Display
  ss2Pdcf : Display
  ss2VdcLINKf : Display
  ss2VdcNEGf : Display
  ss2VdcPOSf : Display
  wires:
  In12/1 -> [ss2Pdcf]
  In1/1 -> [ss1VdcPOSf]
  In3/1 -> [ss1VdcLINKf]
  In2/1 -> [ss1VdcNEGf]
  In4/1 -> [ss1IdcPOSf]
  In6/1 -> [ss1Pdcf]
  In5/1 -> [ss1IdcNEGf]
  In7/1 -> [ss2VdcPOSf]
  In8/1 -> [ss2VdcNEGf]
  In9/1 -> [ss2VdcLINKf]
  In10/1 -> [ss2IdcPOSf]
  In11/1 -> [ss2IdcNEGf]
  [ss1VdcPOSf] -> Mux/1  "ss1VdcPOSf"
  [ss2VdcPOSf] -> Mux/2  "ss2VdcPOSf"
  Mux/1 -> Vdc POS/1
  [ss1VdcPOSf] -> ss1VdcPOSf/1
  [ss2VdcPOSf] -> ss2VdcPOSf/1
  [ss1VdcNEGf] -> Mux1/1  "ss1VdcNEGf"
  [ss2VdcNEGf] -> Mux1/2  "ss2VdcNEGf"
  Mux1/1 -> Vdc NEG/1
  [ss1VdcNEGf] -> ss1VdcNEGf/1
  [ss2VdcNEGf] -> ss2VdcNEGf/1
  [ss1VdcLINKf] -> Mux2/1  "ss1VdcLINKf"
  Mux2/1 -> Vdc LINK/1
  [ss1VdcLINKf] -> ss1VdcLINKf/1
  [ss2VdcLINKf] -> ss2VdcLINKf/1
  [ss2VdcLINKf] -> Mux2/2  "ss2VdcLINKf"
  [ss1IdcPOSf] -> Mux3/1  "ss1IdcPOSf"
  Mux3/1 -> Idc POS/1
  [ss1IdcPOSf] -> ss1IdcPOSf/1
  [ss2IdcPOSf] -> ss2IdcPOSf/1
  [ss2IdcPOSf] -> Mux3/2  "ss2IdcPOSf"
  [ss1IdcNEGf] -> Mux4/1  "ss1IdcNEGf"
  Mux4/1 -> Idc NEG/1
  [ss1IdcNEGf] -> ss1IdcNEGf/1
  [ss2IdcNEGf] -> ss2IdcNEGf/1
  [ss2IdcNEGf] -> Mux4/2  "ss2IdcNEGf"
  Mux5/1 -> Pdc/1
  [ss1Pdcf] -> Mux5/1  "ss1Pdcf"
  [ss2Pdcf] -> Mux5/2  "ss2Pdcf"
  [ss1Pdcf] -> ss1Pdcf/1
  [ss2Pdcf] -> ss2Pdcf/1

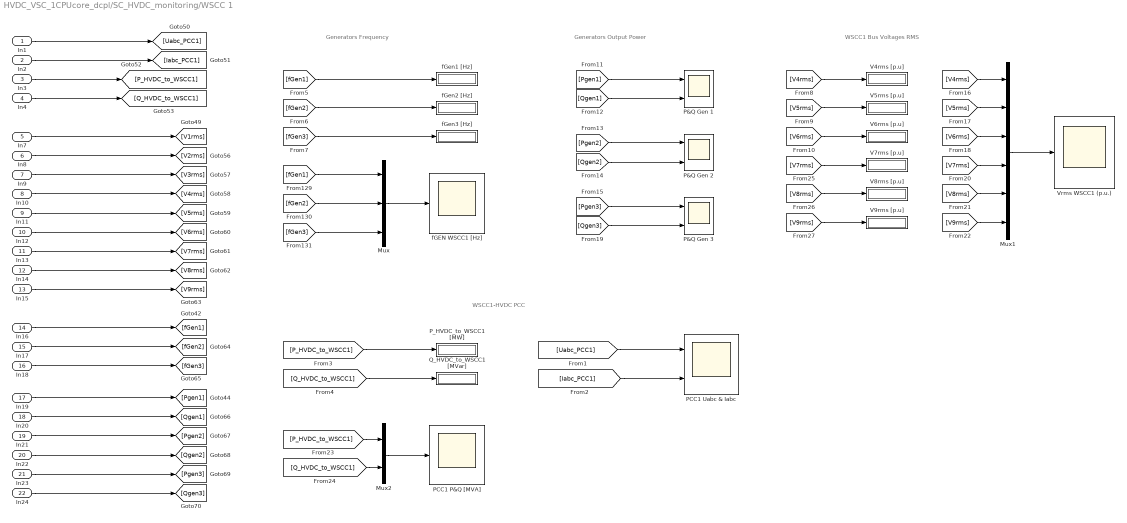
== system HVDC_VSC_1CPUcore_dcpl/SC_HVDC_monitoring/WSCC 1 ==
  note: Generators Frequency
  note: Generators Output Power
  note: WSCC1 Bus Voltages RMS
  note: WSCC1-HVDC PCC
  In1 : Inport
  In2 : Inport  Port=2
  In3 : Inport  Port=3
  In4 : Inport  Port=4
  In7 : Inport  Port=5
  In8 : Inport  Port=6
  In9 : Inport  Port=7
  In10 : Inport  Port=8
  In11 : Inport  Port=9
  In12 : Inport  Port=10
  In13 : Inport  Port=11
  In14 : Inport  Port=12
  In15 : Inport  Port=13
  In16 : Inport  Port=14
  In17 : Inport  Port=15
  In18 : Inport  Port=16
  In19 : Inport  Port=17
  In20 : Inport  Port=18
  In21 : Inport  Port=19
  In22 : Inport  Port=20
  In23 : Inport  Port=21
  In24 : Inport  Port=22
  Mux : Mux  Inputs=3
  Mux1 : Mux  Inputs=6
  Mux2 : Mux  Inputs=2
  P&Q Gen 1 : Scope  NumInputPorts=2
      settings: YMin=6e+07~-1.5e+08  YMax=2.2e+08~2e+08  SaveName=ScopeData19  Decimation=10
  P&Q Gen 2 : Scope  NumInputPorts=2
      settings: YMin=1.626e+08~5.9e+06  YMax=1.642e+08~6.7e+06  SaveName=ScopeData20  Decimation=10
  P&Q Gen 3 : Scope  NumInputPorts=2
      settings: YMin=8.46e+07~-1.115e+07  YMax=8.58e+07~-1.065e+07  SaveName=ScopeData22  Decimation=10
  PCC1 P&Q [MVA] : Scope
      settings: ShowLegends=on  YMin=-2.5e+08  YMax=2.5e+08  SaveName=ScopeData23  Decimation=10
  PCC1 Uabc & Iabc : Scope  NumInputPorts=2
      settings: ShowLegends=on  YMin=-2.5e+08~-5  YMax=2.5e+08~5  SaveName=ScopeData10  Decimation=10
  P_HVDC_to_WSCC1 [MW] : Display
  Q_HVDC_to_WSCC1 [MVar] : Display
  V4rms [p.u] : Display
  V5rms [p.u] : Display
  V6rms [p.u] : Display
  V7rms [p.u] : Display
  V8rms [p.u] : Display
  V9rms [p.u] : Display
  Vrms WSCC1 (p.u.) : Scope
      settings: ShowLegends=on  YMin=0.6  YMax=1.8  SaveName=ScopeData24  Decimation=10
  fGEN WSCC1 [Hz] : Scope
      settings: YMin=59.86  YMax=60.02  SaveName=ScopeData25  Decimation=10
  fGen1 [Hz] : Display
  fGen2 [Hz] : Display
  fGen3 [Hz] : Display
  wires:
  [Qgen2] -> P&Q Gen 2/2
  [Pgen2] -> P&Q Gen 2/1
  [Qgen3] -> P&Q Gen 3/2
  [Pgen3] -> P&Q Gen 3/1
  [Qgen1] -> P&Q Gen 1/2
  [Pgen1] -> P&Q Gen 1/1
  Mux/1 -> fGEN WSCC1 [Hz]/1
  In3/1 -> [P_HVDC_to_WSCC1]
  In10/1 -> [V4rms]
  In15/1 -> [V9rms]
  In12/1 -> [V6rms]
  [P_HVDC_to_WSCC1] -> Mux2/1
  In7/1 -> [V1rms]
  In13/1 -> [V7rms]
  In14/1 -> [V8rms]
  [V6rms] -> Mux1/3
  In8/1 -> [V2rms]
  [fGen1] -> Mux/1
  [V8rms] -> Mux1/5
  Mux2/1 -> PCC1 P&Q [MVA]/1
  In4/1 -> [Q_HVDC_to_WSCC1]
  [V4rms] -> Mux1/1
  In1/1 -> [Uabc_PCC1]
  [V5rms] -> Mux1/2
  In2/1 -> [Iabc_PCC1]
  In11/1 -> [V5rms]
  [V9rms] -> Mux1/6
  [V7rms] -> Mux1/4
  Mux1/1 -> Vrms WSCC1 (p.u.)/1
  [fGen2] -> Mux/2
  [fGen3] -> Mux/3
  In9/1 -> [V3rms]
  [Q_HVDC_to_WSCC1] -> Mux2/2
  In24/1 -> [Qgen3]
  In16/1 -> [fGen1]
  In23/1 -> [Pgen3]
  In19/1 -> [Pgen1]
  In18/1 -> [fGen3]
  In17/1 -> [fGen2]
  In20/1 -> [Qgen1]
  In21/1 -> [Pgen2]
  In22/1 -> [Qgen2]
  [Uabc_PCC1] -> PCC1 Uabc & Iabc/1
  [Iabc_PCC1] -> PCC1 Uabc & Iabc/2
  [fGen1] -> fGen1 [Hz]/1
  [fGen2] -> fGen2 [Hz]/1
  [fGen3] -> fGen3 [Hz]/1
  [V4rms] -> V4rms [p.u]/1
  [V5rms] -> V5rms [p.u]/1
  [V6rms] -> V6rms [p.u]/1
  [V7rms] -> V7rms [p.u]/1
  [V8rms] -> V8rms [p.u]/1
  [V9rms] -> V9rms [p.u]/1
  [P_HVDC_to_WSCC1] -> P_HVDC_to_WSCC1 [MW]/1
  [Q_HVDC_to_WSCC1] -> Q_HVDC_to_WSCC1 [MVar]/1
